simulink model "UAV_Sim"  (R2021b)
settings: Solver=VariableStepAuto  StartTime=0.0  StopTime=30  RelTol=1e-3
settings Model: Creator=Kevin  LastModifiedBy=Kevin

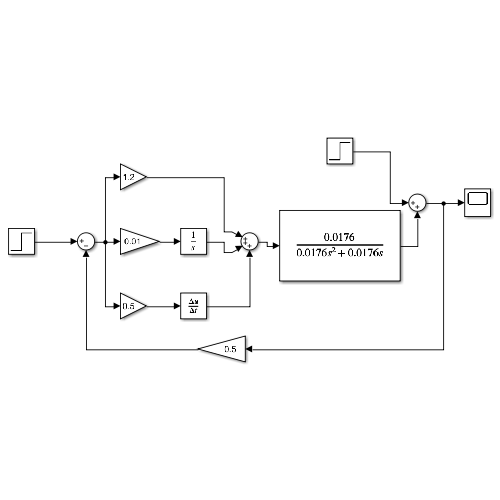
[thumbnail: Simulink's stored preview of the top-level diagram]
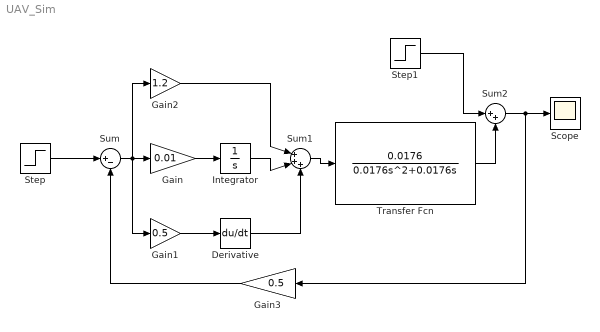
== system UAV_Sim ==
  Derivative : Derivative
  Gain : Gain  Gain=0.01
  Gain1 : Gain  Gain=0.5
  Gain2 : Gain  Gain=1.2
  Gain3 : Gain  Gain=0.5
  Integrator : Integrator
  Scope : Scope
  Step : Step  SampleTime=0
  Step1 : Step  After=0.005  SampleTime=0
  Sum : Sum  Inputs=|+-
  Sum1 : Sum  Inputs=|+++
  Sum2 : Sum  Inputs=|++
  Transfer Fcn : TransferFcn  Numerator=[0.0176]  Denominator=[0.0176 0.0176 0]
  wires:
  Step/1 -> Sum/1
  Gain/1 -> Integrator/1
  Gain2/1 -> Sum1/1
  Integrator/1 -> Sum1/2
  Derivative/1 -> Sum1/3
  Gain1/1 -> Derivative/1
  Gain3/1 -> Sum/2
  Transfer Fcn/1 -> Sum2/2
  Sum2/1 -> Gain3/1, Scope/1
  Step1/1 -> Sum2/1
  Sum1/1 -> Transfer Fcn/1
  Sum/1 -> Gain1/1, Gain2/1, Gain/1
